simulink model "PID"  (R2024b)
settings: Solver=VariableStepAuto  StartTime=0.0  StopTime=10.0  RelTol=1e-3
settings Model: Creator=Shreesha Kumar  LastModifiedBy=Shreesha Kumar

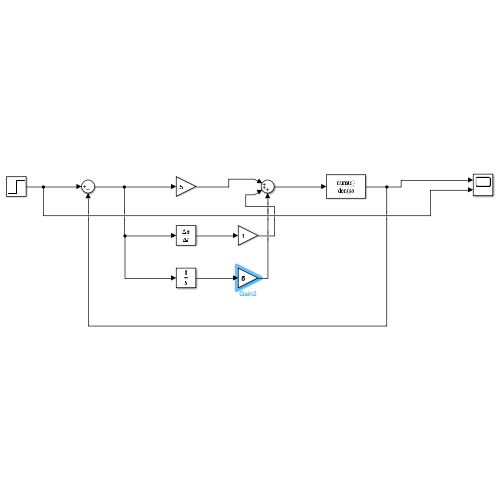
[thumbnail: Simulink's stored preview of the top-level diagram]
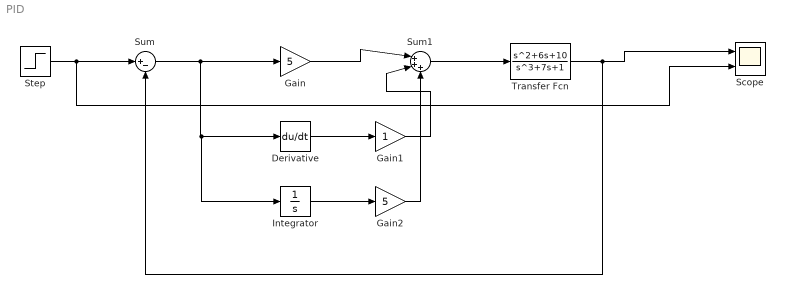
== system PID ==
  Derivative : Derivative
  Gain : Gain  Gain=5
  Gain1 : Gain
  Gain2 : Gain  Gain=5
  Integrator : Integrator
  Scope : Scope  NumInputPorts=2
  Step : Step  SampleTime=0
  Sum : Sum  Inputs=|+-
  Sum1 : Sum  Inputs=|+++
  Transfer Fcn : TransferFcn  Numerator=[1 6 10]  Denominator=[1 ,0,7,1]
  wires:
  Gain/1 -> Sum1/1
  Gain1/1 -> Sum1/2
  Transfer Fcn/1 -> Scope/1, Sum/2
  Derivative/1 -> Gain1/1
  Step/1 -> Sum/1, Scope/2
  Sum1/1 -> Transfer Fcn/1
  Sum/1 -> Integrator/1, Derivative/1, Gain/1
  Gain2/1 -> Sum1/3
  Integrator/1 -> Gain2/1
